simulink model "Domotic_Simulation"  (R2017a)
settings: Solver=ode45  StartTime=0.0  StopTime=Inf  RelTol=1e-3  EnableMultiTasking=on
libraries: fuzblock x1
settings Model: FPTRunName=Active  Creator=The MathWorks, Inc.  LastModifiedBy=juanje
settings DataIOCC: LimitDataPoints=on  SaveFormat=Array
settings OptimizationCC: ExpressionDepthLimit=2147483647  LifeSpan=inf
settings DebuggingCC: UnderspecifiedInitializationDetection=Classic  MergeDetectMultiDrivingBlocksExec=none  FcnCallInpInsideContextMsg=warning  StateNameClashWarn=warning  SFUnexpectedBacktrackingDiag=warning  SFNoUnconditionalDefaultTransitionDiag=warning  SFExecutionAtInitializationDiag=none
settings HardwareCC: ProdBitPerPointer=32  ProdBitPerSizeT=32  ProdBitPerPtrDiffT=32  ProdLargestAtomicFloat=None  ProdIntDivRoundTo=Undefined  ProdEndianess=Unspecified  ProdWordSize=32  ProdHWDeviceType=32-bit Generic
settings ModelReferenceCC: PropagateSignalLabelsOutOfModel=off
settings SFSimCC: SimParseCustomCode=off
settings GRTTargetCC: TargetLangStandard=C89/C90 (ANSI)  GeneratePreprocessorConditionals=Disable all  CombineOutputUpdateFcns=off  GRTInterface=on
settings ConfigComp: CovMetricSettings=dw  CovHtmlReporting=on  CovSaveCumulativeToWorkspaceVar=on  CovSaveSingleToWorkspaceVar=on  CovExternalEMLEnable=off

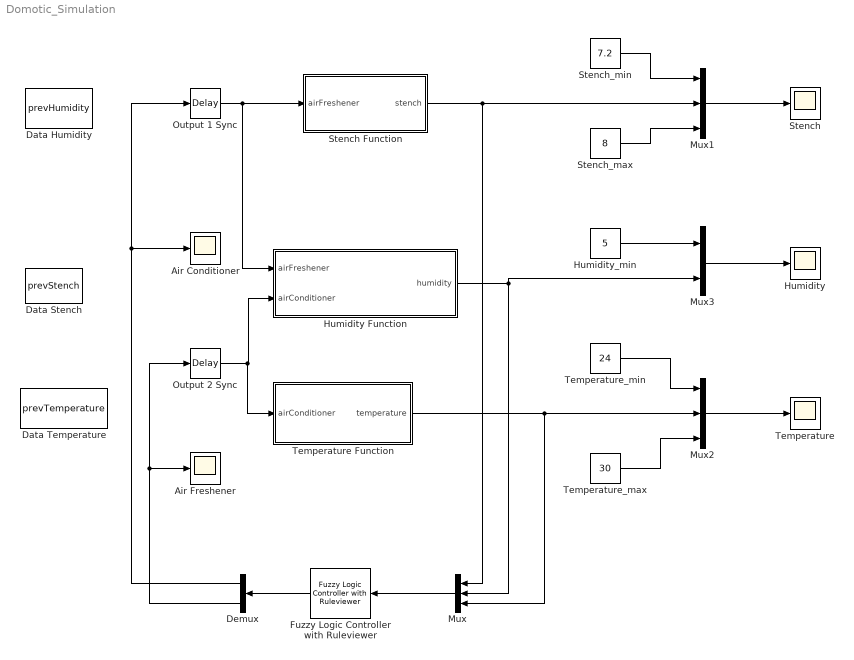
== system Domotic_Simulation ==
  Air Conditioner : Scope
  Air Freshener : Scope
  Data Humidity : DataStoreMemory  DataStoreName=prevHumidity  InitialValue=20  ShowAdditionalParam=off  OutDataTypeStr=double
  Data Stench : DataStoreMemory  DataStoreName=prevStench  InitialValue=2.5  ShowAdditionalParam=off  OutDataTypeStr=double
  Data Temperature : DataStoreMemory  DataStoreName=prevTemperature  InitialValue=25  ShowAdditionalParam=off  OutDataTypeStr=double
  Demux : Demux  Outputs=2
  Fuzzy Logic Controller with Ruleviewer : fuzblock/Fuzzy Logic  Controller  with Ruleviewer  fismatrix=Domotic-controller  Ts=0.1
  Humidity : Scope
  Humidity Function : MATLAB Function  TreatAsAtomicUnit=on
  Humidity_min : Constant  Value=5
  Mux : Mux  Inputs=3
  Mux1 : Mux  Inputs=3
  Mux2 : Mux  Inputs=3
  Mux3 : Mux  Inputs=2
  "Output 1 Sync " : TransportDelay  DelayTime=0.00001
  "Output 2 Sync " : TransportDelay  DelayTime=0.000001
  Stench : Scope
  Stench Function : MATLAB Function  TreatAsAtomicUnit=on
  "Stench_max " : Constant  Value=8
  "Stench_min " : Constant  Value=7.2
  Temperature : Scope
  Temperature Function : MATLAB Function  TreatAsAtomicUnit=on
  Temperature_max : Constant  Value=30
  Temperature_min : Constant  Value=24
  wires:
  "Output 1 Sync "/1 -> Humidity Function/1(airFreshener), Stench Function/1(airFreshener)
  "Stench_min "/1 -> Mux1/1
  Mux1/1 -> Stench/1
  "Stench_max "/1 -> Mux1/3
  Fuzzy Logic Controller with Ruleviewer/1 -> Demux/1
  Demux/1 -> Air Conditioner/1, "Output 1 Sync "/1
  Demux/2 -> Air Freshener/1, "Output 2 Sync "/1
  "Output 2 Sync "/1 -> Temperature Function/1(airConditioner), Humidity Function/2(airConditioner)
  Humidity Function/1(humidity) -> Mux3/2, Mux/2
  Humidity_min/1 -> Mux3/1
  Mux3/1 -> Humidity/1
  Mux/1 -> Fuzzy Logic Controller with Ruleviewer/1
  Stench Function/1(stench) -> Mux/1, Mux1/2
  Temperature Function/1(temperature) -> Mux/3, Mux2/2
  Temperature_min/1 -> Mux2/1
  Mux2/1 -> Temperature/1
  Temperature_max/1 -> Mux2/3

== matlab function Domotic_Simulation/Temperature Function ==
  data: temperature output; prevTemperature data_store_memory; airConditioner input
function temperature = funcionTemp(airConditioner)
%#codegen
global prevTemperature;
Caudal_max=10;

potencia=(airConditioner/100)*Caudal_max;

potencia_parado=(4.8/100)*Caudal_max;
potencia_baja=(27.86/100)*Caudal_max;
potencia_media=(60/100)*Caudal_max;


if potencia<potencia_parado %Caudal Parada
    prevTemperature = prevTemperature+0.5;
end

if potencia>potencia_parado && potencia< potencia_baja % Caudal bajo
    prevTemperature = prevTemperature;
end

if potencia>potencia_baja && potencia < potencia_media %Caudal medio
    prevTemperature = prevTemperature-0.2;
end

if potencia>potencia_media %Caudal Alto
    prevTemperature= prevTemperature-0.5;
end

% Comprobación de que la temperatura no sea negativa


temperature = prevTemperature;

== matlab function Domotic_Simulation/Stench Function ==
  data: stench output; prevHumidity data_store_memory; airFreshener input
function stench = stenchUpdate(airFreshener)
%#codegen
global prevHumidity;
x1 = double(0);
x2 = double(0);
Cloro_max=25;

g_cloro=(airFreshener/100)*Cloro_max;

cloro_nada=(5/100)*Cloro_max;
Volumen_piscina=800000;

%% Dosificador de cloro parado
if g_cloro<cloro_nada
    prevHumidity=prevHumidity+0.5;
end

%% Dosificador de cloro encendido
if g_cloro>cloro_nada
    % Calculo gramos HCl
    g_HCl=g_cloro*1.125*20/100;
    %Cálculo concentración debiado al cloro añadido
    c1=g_HCl/(Volumen_piscina*36.5);
    %Cálculo de la concentración debido al cloro que ya había en la piscina
    c_H3O=10^(-prevHumidity);
     %Cálculo concentración total
    conc=c1+c_H3O;
    %Concentración debido al agua (disolución muy diluida)
    
         %% Ecuacion de segundo grado
         a=1;
         b=conc;
         c=-10E-14;
         d=b^2-4*a*c;
            if d>0
                x1=(-b+sqrt(d))/(2*a);
                x2=(-b-sqrt(d))/(2*a);
    
            elseif d==0
                x1=-b/(2*a);
                x2=x1;
            else 
                disp('d<0 Raiz imaginaria');   
            end
        % Seleccionamos la solucion positiva

            x=max(x1,x2);
  
  %% Cálculo del pH
    prevHumidity=-log10(conc+x);

end
 %% Comprobación de que el valor del pH no sea negativo
if prevHumidity<0
    prevHumidity=0;
end

stench = prevHumidity;

== matlab function Domotic_Simulation/Humidity Function ==
  data: humidity output; prevStench data_store_memory; airFreshener input; airConditioner input
function humidity = humidityUpdate(airFreshener, airConditioner)

global prevStench;

Cloro_max=25;
Caudal_max=10;
g_cloro=(airFreshener/100)*Cloro_max;
potencia=(airConditioner/100)*Caudal_max;


potencia_parado=(4.8/100)*Caudal_max;
potencia_baja=(27.86/100)*Caudal_max;
potencia_media=(60/100)*Caudal_max;

cloro_nada=(5/100)*Cloro_max;
cloro_bajo=(24.7/100)*Cloro_max;
cloro_medio=(65/100)*Cloro_max;

if g_cloro<cloro_nada && potencia<potencia_parado %Cloro nada y caudal parado
        prevStench = prevStench+0.1;
end

if (g_cloro>cloro_nada && g_cloro<cloro_bajo && potencia <potencia_parado)||... %Cloro bajo y caudal parado
    (g_cloro<cloro_nada && potencia>potencia_parado && potencia<potencia_baja) % Cloro nada y caudal bajo 
    
        prevStench = prevStench;
    
end

if (g_cloro>cloro_bajo && g_cloro<cloro_medio && potencia<potencia_parado)||... %Cloro medio y caudal parado
        (g_cloro>cloro_nada && g_cloro<cloro_bajo && potencia>potencia_parado && potencia<potencia_baja)||... %Cloro bajo y caudal bajo
            (g_cloro<cloro_nada && potencia>potencia_baja && potencia<potencia_media) %Cloro nada y caudal medio
        
        prevStench= prevStench-0.1;
end

if (g_cloro>cloro_medio && potencia<potencia_parado)||... %Cloro alto y caudal parado
        (g_cloro<cloro_medio && g_cloro>cloro_bajo && potencia>potencia_parado && potencia<potencia_baja) || ... % Cloro medio y caudal bajo
            (g_cloro<cloro_bajo && g_cloro>cloro_nada && potencia>potencia_baja && potencia<potencia_media) || ... % Cloro bajo y caudal medio
                (g_cloro<cloro_nada && potencia>potencia_media) %Cloro nada y caudal alto
         prevStench = prevStench-0.2;
end

if (g_cloro>cloro_medio && potencia>potencia_parado && potencia<potencia_baja) ||... %Cloro alto y caudal bajo
        (g_cloro>cloro_bajo && g_cloro<cloro_medio && potencia>potencia_baja && potencia<potencia_media) || ... %Cloro medio y caudal medio
            (g_cloro>cloro_nada && g_cloro<cloro_bajo && potencia>potencia_media) %Cloro bajo y caudal alto
        prevStench= prevStench-0.3;
end

if (g_cloro>cloro_medio && potencia>potencia_baja && potencia<potencia_media) ||... %Cloro alto y caudal medio
        (g_cloro>cloro_bajo && g_cloro<cloro_medio && potencia>potencia_media) %Cloro medio y caudal alto
        prevStench = prevStench-0.4;
end

if (g_cloro>cloro_medio && potencia>potencia_media) %Cloro alto y caudal alto
        prevStench = prevStench-0.5;
end

%Comprobación de que la turbidez no sea negativa
if prevStench<0
    prevStench=0;
end

humidity=prevStench;
